simulink model "sldemo_VariableTransportDelay_pipe"  (Simulink 7.6)
settings: Solver=ode45  StartTime=0.0  StopTime=10.0  MaxStep=0.01  RelTol=1e-3
libraries: simulink x2
Description:
  | Incompressible flow through a fixed length pipe
  | 
  | An incompressible flow goes through a pipe of length L with speed v(t).
  | At the inlet the flow temperature is Ti, then the temperature at the
  | outletTo can be modeled as an variable transport delay of  Ti. At time
  | t=0, the pipe is empty and  until t=2, there is no flow at the outlet.
  | Thus the output temperature before t=2 is the initial output temperature.
settings Model: Creator=The MathWorks Inc.  ExtModeAutoUpdateStatusClock=off
settings OptimizationCC: InitFltsAndDblsToZero=on
settings DebuggingCC: SaveWithParameterizedLinksMsg=none  SignalResolutionControl=TryResolveAllWithWarning  MultiTaskDSMMsg=warning  MultiTaskCondExecSysMsg=none
settings RTWCC: IncludeERTFirstTime=on
settings GRTTargetCC: TargetFcnLib=ansi_tfl_tmw.mat

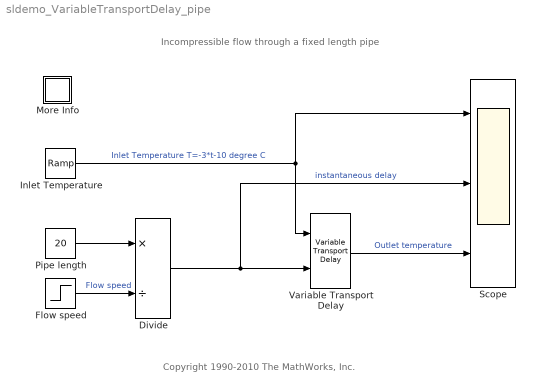
== system sldemo_VariableTransportDelay_pipe ==
  note: Incompressible flow through a fixed length pipe
  note: Copyright 1990-2010 The MathWorks, Inc.
  Divide : Product  Inputs=*/
  Flow speed : Step  Time=5  Before=10  After=20  SampleTime=0
  Inlet Temperature : simulink/Sources/Ramp  SystemSampleTime=-1  slope=3  start=0  X0=-10
  More Info : Subsystem
      settings: OpenFcn=showdemo('sldemo_VariableTransportDelay')
      mask Display: disp('?')
  Pipe length : Constant  Value=20
  Scope : Scope  NumInputPorts=3
      settings: TimeRange=10  YMin=-20~0.5~-20  YMax=20~2.5~20
  Variable Transport Delay : VariableTransportDelay  VariableDelayType=Variable transport delay  MaximumDelay=1000  InitialOutput=-15
  wires:
  Variable Transport Delay/1 -> Scope/3  "Outlet temperature"
  Divide/1 -> Scope/2, Variable Transport Delay/2  "instantaneous delay"
  Flow speed/1 -> Divide/2  "Flow speed"
  Pipe length/1 -> Divide/1
  Inlet Temperature/1 -> Scope/1, Variable Transport Delay/1  "Inlet Temperature T=-3*t-10 degree C"

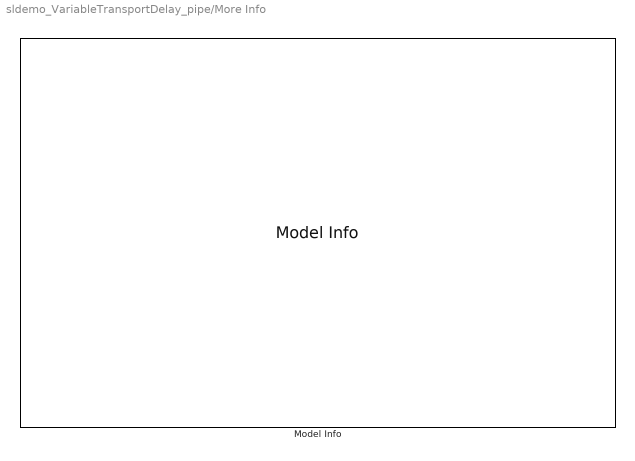
== system sldemo_VariableTransportDelay_pipe/More Info ==
  Model Info : simulink/Model-Wide Utilities/Model Info  InitialBlockCM=None  BlockCM=None  Frame=on  HorizontalTextAlignment=Left  LeftAlignmentValue=0.02  SourceBlockDiagram=sldemo_VariableTransportDelay_pipe  TagMaxNumber=20
